simulink model "VFControl"  (R2024b)
settings: Solver=VariableStepAuto  StartTime=0.0  StopTime=2.5  MaxStep=5e-5  RelTol=1e-3
libraries: spsAsynchronousMachineSIUnitsLib x1, spsDCVoltageSourceLib x1, mcbcontrolslib x1, slpidlib x1, eePwmGeneratorTwoLevel x1, spsUniversalBridgeLib x1, sps_lib x1
settings Model: Creator=joekr  LastModifiedBy=joekr

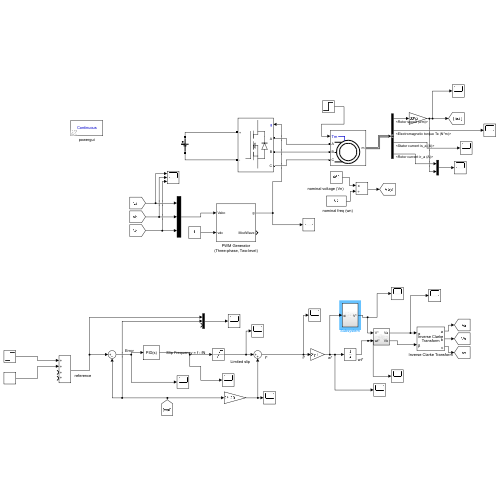
[thumbnail: Simulink's stored preview of the top-level diagram]
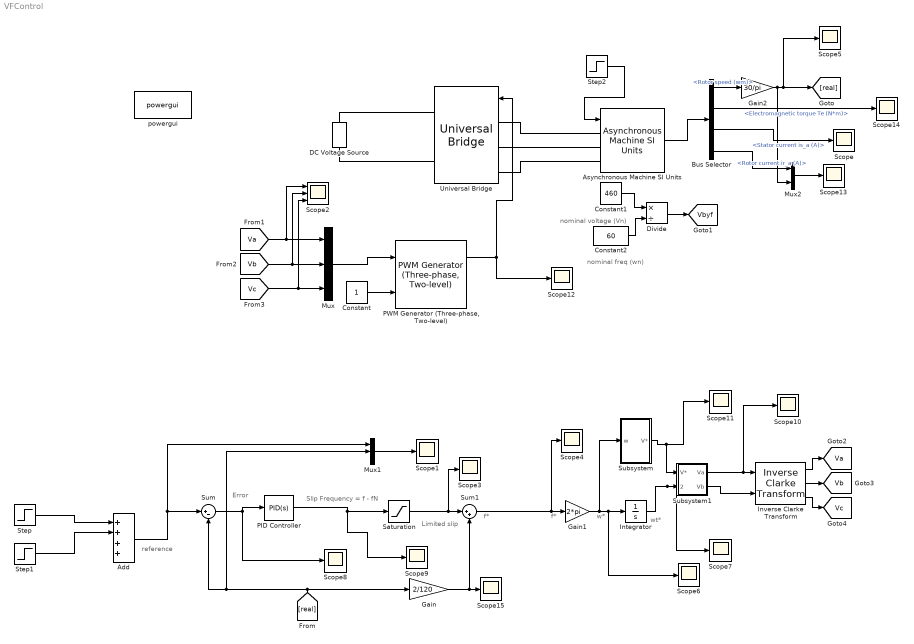
== system VFControl ==
  note: reference
  note: Limited slip
  note: nominal voltage (Vn)
  note: nominal freq (wn)
  note: wt*
  note: w*
  note: f*
  note: Slip Frequency = f - fN
  note: Error
  note: f*
  Add : Sum  Inputs=++++
  Asynchronous Machine SI Units : spsAsynchronousMachineSIUnitsLib/Asynchronous Machine SI Units  RotorType=Squirrel-cage  PresetModel="01:  5 HP   460 V 60Hz 1750 RPM"  MechanicalLoad=Torque Tm  ShowDetailedParameters=on  ReferenceFrame=Rotor  Units=SI  MeasurementBus=off  NominalParameters=[3730 460 60]  VoltageRatio=1  Stator=[1.115 0.005974]  Rotor=[1.083 0.005974]  Cage1=[0.4155 0.002066]  Cage2=[0.4168 0.0003495]  Lm=0.2037  Mechanical=[0.02 0.005752 2]  PolePairs=2  InitialConditions=[0 0 0 0 0 0 0 0]  SimulateSaturation=off  Saturation=[14.03593122, 27.81365428, 53.79336849, 72.68890987, 97.98006896, 148.6815601, 215.7428561, 302.9841135, 428.7778367 ; 230, 322, 414, 460, 506, 552, 598, 644, 690]  LoadFlowParameters=1492000  TsPowergui=0  TsBlock=-1  IterativeModel=Trapezoidal non iterative  IterativeDiscreteModel=Trapezoidal non iterative  Pmec=1.492e+006
  Bus Selector : BusSelector  OutputSignals=Mechanical.Rotor speed (wm),Mechanical.Electromagnetic torque Te (N*m),Stator measurements.Stator current is_a (A),Rotor measurements.Rotor current ir_a (A)
  Constant : Constant  SampleTime=5e-5
  Constant1 : Constant  Value=460  SampleTime=5e-5
  Constant2 : Constant  Value=60  SampleTime=5e-5
  DC Voltage Source : spsDCVoltageSourceLib/DC Voltage Source  Amplitude=650  Measurements=None
  Divide : Product  Inputs=*/
  Gain : Gain  Gain=2/120
  Gain1 : Gain  Gain=2*pi
  Gain2 : Gain  Gain=30/pi
  Integrator : Integrator
  Inverse Clarke Transform : mcbcontrolslib/Inverse Clarke Transform  PhaseInput=Two inputs  EnPowerInv=off
      settings: LibrarySourceBlock=mcbhdllib/Controls/Math Transforms/Inverse Clarke Transform
  Mux : Mux  Inputs=3
  Mux1 : Mux  Inputs=3
  Mux2 : Mux  Inputs=2
  PID Controller : slpidlib/PID Controller  Controller=PID  Form=Parallel  TimeDomain=Continuous-time  UseExternalTs=off  SampleTime=-1  IntegratorMethod=Forward Euler  FilterMethod=Forward Euler  ControllerParametersSource=internal  P=0.008  I=0.35  UseKiTs=off  D=0.00013  UseExternalDerivativeSource=off  N=100  UseFilter=on  TunerSelectOption=Transfer Function Based (PID Tuner App)  InitialConditionSource=internal  InitialConditionForIntegrator=0  InitialConditionForFilter=0  DifferentiatorICPrevScaledInput=0  ExternalReset=none  TrackingMode=off  Kt=1  LimitOutput=off  SatLimitsSource=internal  UpperSaturationLimit=inf  LowerSaturationLimit=-inf  LinearizeAsGain=on  AntiWindupMode=none  Kb=1  LimitIntegrator=off  UpperIntegratorSaturationLimit=inf  LowerIntegratorSaturationLimit=-inf  POutMin=[]  POutMax=[]  IOutMin=[]  IOutMax=[]  DOutMin=[]  DOutMax=[]  NOutMin=[]  NOutMax=[]  SumOutMin=[]  SumOutMax=[]  SaturationOutMin=[]  SaturationOutMax=[]  PParamMin=[]  PParamMax=[]  IParamMin=[]  IParamMax=[]  DParamMin=[]  DParamMax=[]  NParamMin=[]  NParamMax=[]  KbParamMin=[]  KbParamMax=[]  KtParamMin=[]  KtParamMax=[]  KbOutMin=[]  KbOutMax=[]  KtOutMin=[]  KtOutMax=[]  IntegratorOutMin=[]  IntegratorOutMax=[]  FilterOutMin=[]  FilterOutMax=[]  SumI1OutMin=[]  SumI1OutMax=[]  SumI2OutMin=[]  SumI2OutMax=[]  SumI3OutMin=[]  SumI3OutMax=[]  SumI4OutMin=[]  SumI4OutMax=[]  SumDOutMin=[]  SumDOutMax=[]  DifferentiatorOutMin=[]  DifferentiatorOutMax=[]  FilterDiffOutCoefMin=[]  FilterDiffOutCoefMax=[]  ReciprocalOutMin=[]  ReciprocalOutMax=[]  SumDenOutMin=[]  SumDenOutMax=[]  SumNumOutMin=[]  SumNumOutMax=[]  DivideOutMin=[]  DivideOutMax=[]  UdiffTsProdOutMin=[]  UdiffTsProdOutMax=[]  NTsProdOutMin=[]  NTsProdOutMax=[]  UintegralTsProdOutMin=[]  UintegralTsProdOutMax=[]  UngainTsProdOutMin=[]  UngainTsProdOutMax=[]  ClampingZeroOutDataTypeStr=Inherit: Inherit via back propagation  ClampingZeroOutMin=[]  ClampingZeroOutMax=[]  FilterDenConstantOutDataTypeStr=Inherit: Inherit via back propagation  FilterDenConstantOutMin=[]  FilterDenConstantOutMax=[]  PCopyOutDataTypeStr=Inherit: Inherit via back propagation  PCopyOutMin=[]  PCopyOutMax=[]  NCopyOutDataTypeStr=Inherit: Inherit via back propagation  NCopyOutMin=[]  NCopyOutMax=[]  IntegratorContinuousStateAttributes=''  IntegratorStateMustResolveToSignalObject=off  IntegratorRTWStateStorageClass=Auto  FilterContinuousStateAttributes=''  FilterStateMustResolveToSignalObject=off  FilterRTWStateStorageClass=Auto  ParallelPVariant=InternalParameters  IdealPVariant=Disabled  IVariant=InternalParameters  DVariant=InternalParameters  IntegratorVariant=Continuous  SatVariant=Disabled  AWVariant=Passthrough  PCopyVariant=Disabled  TRVariant=Disabled  FdbkBlocksVariant=Forward  IdealPFdbkVariant=Disabled  SatFdbkVariant=Disabled  DerivativeFilterVariant=ContFilter  NVariant=InternalParameters  NCopyVariant=Disabled  FilterICVariant=InternalICsFilter  IntegratorICVariant=InternalICs  ExternalResetVariant=Disabled  TRSumVariant=Passthrough  SumFdbkVariant=Disabled  SumVariant=Sum_PID  TsampFilterVariant=InternalTs  TsampNgainVariant=Passthrough  TsampIntegralVariant=Disabled_SignalSpec  ExternalSaturationOutDataTypeStr=Inherit: Same as second input  DerivativeSourceVariant=ErrorSignal  PreIntVariant=InternalPreInt
  "PWM Generator (Three-phase, Two-level)" : eePwmGeneratorTwoLevel/PWM Generator (Three-phase, Two-level)  PWMMode=Continuous PWM (CPWM)  CPWMMode=SPWM: sinusoidal PWM  DPWMMode=60 DPWM: 60 degree discontinuous PWM  fsw=1000  Ts=5e-5
      settings: LibrarySourceBlock=|
      | ee_sl_lib/Pulse Width
      | Modulation/PWM Generator
      | (Three-phase, Two-level)
  Saturation : Saturate  UpperLimit=60  LowerLimit=0
  Scope{,1,3..15} (15 alike) : Scope
  Scope2 : Scope  NumInputPorts=3
  Step : Step  Time=0.5  After=1000  SampleTime=0
  Step1 : Step  After=500  SampleTime=0
  Step2 : Step  Time=1.5  After=100  SampleTime=5e-5
  Subsystem : Subsystem
  Subsystem1 : Subsystem
  Sum : Sum  Inputs=|+-
  Sum1 : Sum  Inputs=|++
  Universal Bridge : spsUniversalBridgeLib/Universal Bridge  Arms=3  SnubberResistance=1e5  SnubberCapacitance=inf  Device=MOSFET / Diodes  Ron=1e-3  Lon=0  ForwardVoltages="[  0  0  ]"  ForwardVoltage=0  GTOparameters=[ 10e-6 , 20e-6 ]  IGBTparameters=[ 1e-6 , 2e-6 ]  Measurements=None  Measurements_2=None  converterType=Rectifier
  powergui : sps_lib/powergui  Priority=1  SimulationMode=Continuous  SampleTime=50e-6  frequency=60  Iterations=50  frequencyindice=60  Pbase=100e6  ErrMax=1e-4  UnitsV=kV  UnitsW=MW  buscounter=0  FunctionMessages=off  echomessages=off  EnableUseOfTLC=off  CurrentSourceSwitches=off  DisableSnubberDevices=off  DisableRonSwitches=off  DisableVfSwitches=off  DisplayEquations=off  AutomaticDiscreteSolvers=off  SolverType=Tustin/Backward Euler (TBE)  Interpol=off  ExternalGateDelay=off  methode=off  Ts=100  x0status=blocks  SPID=on  SwTol=0  HookPort=off  NonlinearTolerance=1e-4  nMaxIteration=100  ContinueOnMaxIteration=off  RestoreLinks=warning  ResistiveCurrentMeasurement=off  Frange=[0:2:500]  Ylog=off  Xlog=on  ShowGrid=off  save=off  variable=ZData  structure=0  ZoomFFT=off  StartTime=0.0  cycles=1  DisplayStyle=1  fundamental=60  FreqAxis=off  MaxFrequency=1000  frequencyindicesteady=1  RmsSteady=1  display=off
  tag scope: Va=global, Vb=global, Vbyf=global, Vc=global
  wires:
  Asynchronous Machine SI Units/1 -> Bus Selector/1
  Mux/1 -> "PWM Generator (Three-phase, Two-level)"/1
  "PWM Generator (Three-phase, Two-level)"/1 -> Universal Bridge/1, Scope12/1
  Constant/1 -> "PWM Generator (Three-phase, Two-level)"/2
  [real] -> Gain/1, Mux1/2, Sum/2
  Sum/1 -> Scope8/1, PID Controller/1
  Saturation/1 -> Scope3/1, Sum1/1
  Gain/1 -> Scope15/1, Sum1/2
  Sum1/1 -> Scope4/1, Gain1/1
  Gain1/1 -> Scope6/1, Integrator/1, Subsystem/1(w)
  Constant1/1 -> Divide/1
  Constant2/1 -> Divide/2
  Divide/1 -> [Vbyf]
  Integrator/1 -> Scope7/1, Subsystem1/2(wt*)
  Subsystem/1(V*) -> Scope11/1, Subsystem1/1(V*)
  Subsystem1/2(Vb) -> Inverse Clarke Transform/2
  Subsystem1/1(Va) -> Scope10/1, Inverse Clarke Transform/1
  Inverse Clarke Transform/2 -> [Vb]
  Inverse Clarke Transform/3 -> [Vc]
  Inverse Clarke Transform/1 -> [Va]
  [Va] -> Scope2/1, Mux/1
  [Vb] -> Scope2/2, Mux/2
  [Vc] -> Scope2/3, Mux/3
  Bus Selector/2 -> Scope14/1  "<Electromagnetic torque Te (N*m)>"
  Step/1 -> Add/1
  Add/1 -> Mux1/1, Sum/1
  Step2/1 -> Asynchronous Machine SI Units/1
  Bus Selector/3 -> Scope/1  "<Stator current is_a (A)>"
  Bus Selector/1 -> Gain2/1  "<Rotor speed (wm)>"
  Gain2/1 -> Mux2/2, Scope5/1, [real]
  PID Controller/1 -> Scope9/1, Saturation/1
  Mux1/1 -> Scope1/1
  Mux2/1 -> Scope13/1
  Bus Selector/4 -> Mux2/1  "<Rotor current ir_a (A)>"
  Step1/1 -> Add/2
  connections:
  DC Voltage Source/RConn1 -- Universal Bridge/RConn1
  DC Voltage Source/LConn1 -- Universal Bridge/RConn2
  Universal Bridge/LConn2 -- Asynchronous Machine SI Units/LConn2
  Universal Bridge/LConn3 -- Asynchronous Machine SI Units/LConn3
  Universal Bridge/LConn1 -- Asynchronous Machine SI Units/LConn1

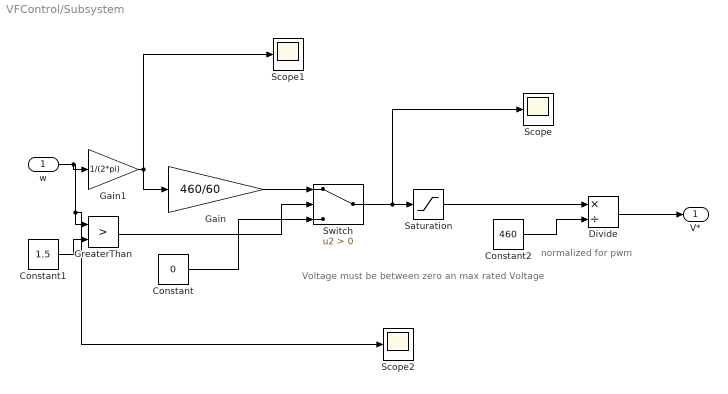
== system VFControl/Subsystem ==
  note: normalized for pwm
  note: Voltage must be between zero an max rated Voltage
  w : Inport
  Constant : Constant  Value=0  SampleTime=5e-5
  Constant1 : Constant  Value=1.5  SampleTime=5e-5
  Constant2 : Constant  Value=460  SampleTime=5e-5
  Divide : Product  Inputs=*/
  Gain : Gain  Gain=460/60
  Gain1 : Gain  Gain=1/(2*pi)
  GreaterThan : RelationalOperator  Operator=>  OutDataTypeStr=boolean  RndMeth=Simplest  InputSameDT=off
  Saturation : Saturate  UpperLimit=460  LowerLimit=0
  Scope : Scope
  Scope1 : Scope
  Scope2 : Scope
  Switch : Switch  Criteria=u2 > Threshold  SaturateOnIntegerOverflow=off  InputSameDT=off
  V* : Outport
  wires:
  w/1 -> Gain1/1, Scope2/1, GreaterThan/1
  Switch/1 -> Scope/1, Saturation/1
  Gain/1 -> Switch/1
  Constant/1 -> Switch/3
  GreaterThan/1 -> Switch/2
  Constant1/1 -> GreaterThan/2
  Gain1/1 -> Scope1/1, Gain/1
  Saturation/1 -> Divide/1
  Divide/1 -> V*/1
  Constant2/1 -> Divide/2

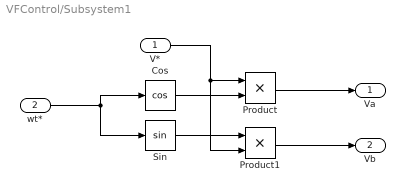
== system VFControl/Subsystem1 ==
  V* : Inport
  wt* : Inport  Port=2
  Cos : Trigonometry  Operator=cos
  Product : Product
  Product1 : Product
  Sin : Trigonometry
  Va : Outport
  Vb : Outport  Port=2
  wires:
  Product/1 -> Va/1
  Product1/1 -> Vb/1
  V*/1 -> Product1/2, Product/1
  wt*/1 -> Sin/1, Cos/1
  Sin/1 -> Product1/1
  Cos/1 -> Product/2
